simulink model "modelling_nl"  (R2024b)
settings: Solver=VariableStepAuto  StartTime=0.0  StopTime=sim_nl.t  RelTol=1e-3
values from neighbouring files (symbols this model uses):
  params = parameters()    [mainfile_nl.m]
undefined symbols (not defined in the file or in its folder): nl_model
settings Model: Creator=ben83  LastModifiedBy=ben
settings RTWCC: GPUComputeCapability=3.5

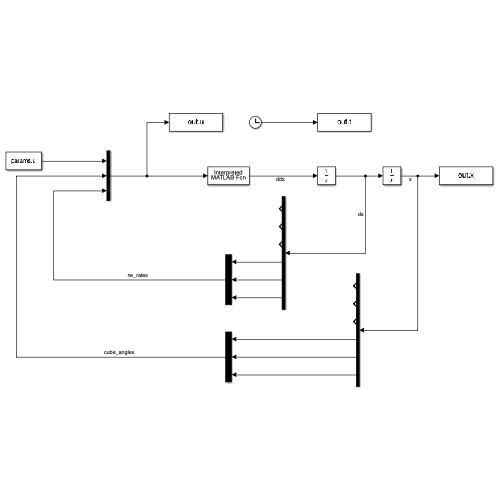
[thumbnail: Simulink's stored preview of the top-level diagram]
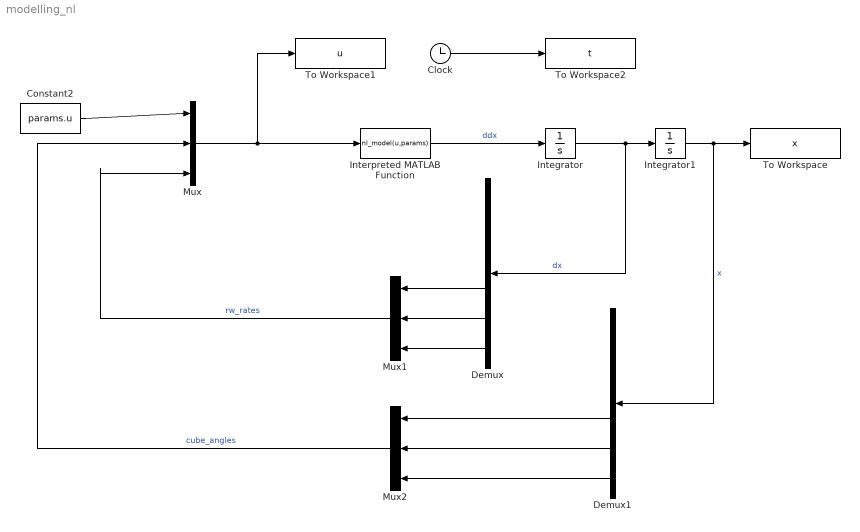
== system modelling_nl ==
  Clock : Clock
  Constant2 : Constant  Value=params.u
  Demux : Demux  Outputs=6
  Demux1 : Demux  Outputs=6
  Integrator : Integrator  InitialCondition=params.ic_rates
  Integrator1 : Integrator  InitialCondition=params.ic_vel
  Interpreted MATLAB Function : MATLABFcn  MATLABFcn=nl_model(u,params)
  Mux : Mux  Inputs=3
  Mux1 : Mux  Inputs=3
  Mux2 : Mux  Inputs=3
  To Workspace : ToWorkspace  VariableName=x  SampleTime=-1
  To Workspace1 : ToWorkspace  VariableName=u  SampleTime=-1
  To Workspace2 : ToWorkspace  VariableName=t  SampleTime=-1
  wires:
  Interpreted MATLAB Function/1 -> Integrator/1  "ddx"
  Mux/1 -> To Workspace1/1, Interpreted MATLAB Function/1
  Clock/1 -> To Workspace2/1
  Constant2/1 -> Mux/1
  Integrator/1 -> Demux/1, Integrator1/1  "dx"
  Integrator1/1 -> Demux1/1, To Workspace/1  "x"
  Demux/5 -> Mux1/2
  Demux/6 -> Mux1/3
  Demux/4 -> Mux1/1
  Demux1/4 -> Mux2/1
  Demux1/5 -> Mux2/2
  Demux1/6 -> Mux2/3
  Mux2/1 -> Mux/2  "cube_angles"
  Mux1/1 -> Mux/3  "rw_rates"
